simulink model "untitled"  (R2026a)
settings: Solver=VariableStepAuto  StopTime=100
settings Model: Creator=Lenovo  LastModifiedBy=Lenovo

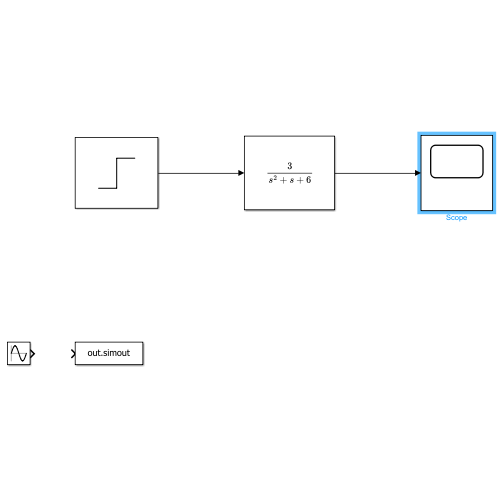
[thumbnail: Simulink's stored preview of the top-level diagram]
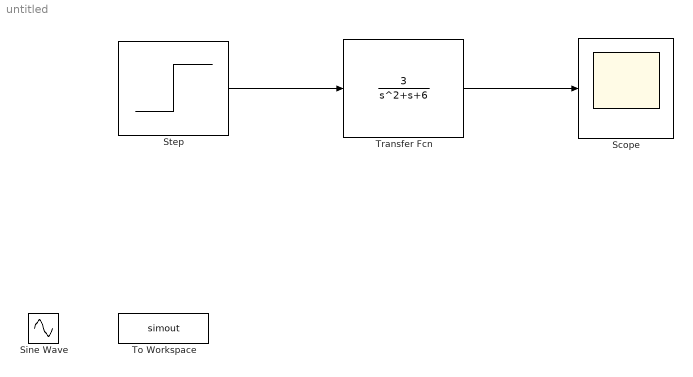
== system untitled ==
  Scope : Scope
      settings: ActiveDisplayYMinimum=-0.093353131343657622  ActiveDisplayYMaximum=0.84017818209291872
  Sine Wave : Sin  SampleTime=0
  Step : Step  SampleTime=0
  To Workspace : ToWorkspace  VariableName=simout  SampleTime=-1
  Transfer Fcn : TransferFcn  Numerator=[3]  Denominator=[1 1 6]
  wires:
  Step/1 -> Transfer Fcn/1
  Transfer Fcn/1 -> Scope/1
